simulink model "FirstOrderSystemSimulinkRL"  (R2019b)
settings: Solver=VariableStepAuto  StartTime=0.0  StopTime=25  RelTol=1e-1
values from neighbouring files (symbols this model uses):
  Ts = 0.05    [FirstOrderSystemScriptDQN.m]    (also in Trained Data Workspace.mat)
undefined symbols (not defined in the file or in its folder): DiscIntNeverNeededParam
libraries: simulink x4, dspswit3 x2, rllib x1
settings Model: Creator=PC  LastModifiedBy=PC

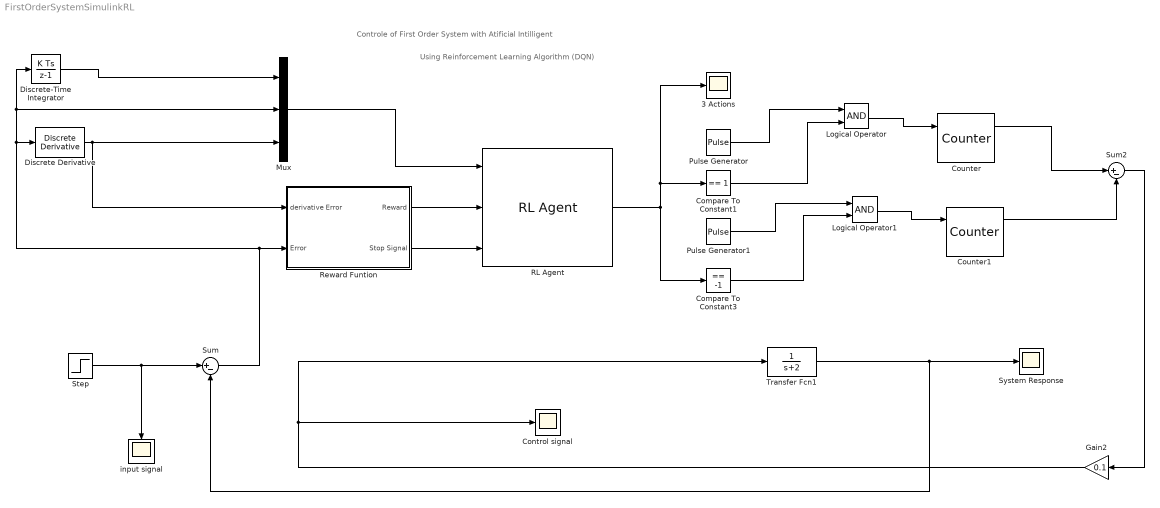
== system FirstOrderSystemSimulinkRL ==
  note: Using Reinforcement Learning Algorithm (DQN)
  note: Controle of First Order System with Atificial Intilligent
  3 Actions : Scope
  Compare To Constant1 : simulink/Logic and Bit Operations/Compare To Constant  relop===  const=1  OutDataTypeStr=boolean
  Compare To Constant3 : simulink/Logic and Bit Operations/Compare To Constant  relop===  const=-1  OutDataTypeStr=boolean
  Control signal : Scope
  Counter : dspswit3/Counter  Direction=Up  CountEvent=Rising edge  CounterSize=User defined  MaxCount=1000  InitialCount=0  Output=Count and Hit  HitValue=32  ResetInput=on  SamplesPerFrame=1  Ts=1  CntDtype=double  HitDtype=Logical
  Counter1 : dspswit3/Counter  Direction=Up  CountEvent=Rising edge  CounterSize=User defined  MaxCount=1000  InitialCount=0  Output=Count and Hit  HitValue=32  ResetInput=on  SamplesPerFrame=1  Ts=1  CntDtype=double  HitDtype=Logical
  Discrete Derivative : simulink/Discrete/Discrete Derivative  gainval=1.0  ICPrevScaledInput=0.0  OutMin=[]  OutMax=[]  OutDataType=fixdt(1, 16)  OutScaling=2^-10  DoSatur=off
  Discrete-Time Integrator : DiscreteIntegrator  SampleTime=Ts  ICPrevOutput=DiscIntNeverNeededParam  ICPrevScaledInput=DiscIntNeverNeededParam
  Gain2 : Gain  Gain=0.1
  Logical Operator : Logic  AllPortsSameDT=off  OutDataTypeStr=boolean
  Logical Operator1 : Logic  AllPortsSameDT=off  OutDataTypeStr=boolean
  Mux : Mux  Inputs=3
  Pulse Generator : DiscretePulseGenerator  PulseType=Time based  Period=0.1  PulseWidth=0.05
  Pulse Generator1 : DiscretePulseGenerator  PulseType=Time based  Period=0.1  PulseWidth=0.05
  RL Agent : rllib/RL Agent  Agent=agent  ProvideReward=on  ProvideIsDone=on  ProvideCumRwd=off  TreatAsDirectFeedthrough=on  CollectLoggedSignals=on  CollectModelStates=on
      settings: SourceProductName=Reinforcement Learning Toolbox
  Reward Funtion : Subsystem
  Step : Step  Time=0  SampleTime=0
  Sum : Sum  Inputs=|+-
  Sum2 : Sum  Inputs=|+-
  System Response : Scope
  Transfer Fcn1 : TransferFcn  Denominator=[1 2]
  input signal : Scope
  wires:
  Step/1 -> Sum/1, input signal/1
  Sum/1 -> Reward Funtion/2(Error), Discrete-Time Integrator/1, Mux/2, Discrete Derivative/1
  Discrete-Time Integrator/1 -> Mux/1
  Discrete Derivative/1 -> Reward Funtion/1(derivative Error), Mux/3
  Mux/1 -> RL Agent/1
  RL Agent/1 -> 3 Actions/1, Compare To Constant1/1, Compare To Constant3/1
  Pulse Generator/1 -> Logical Operator/1
  Logical Operator/1 -> Counter/1
  Compare To Constant1/1 -> Logical Operator/2
  Compare To Constant3/1 -> Logical Operator1/2
  Logical Operator1/1 -> Counter1/1
  Pulse Generator1/1 -> Logical Operator1/1
  Counter/1 -> Sum2/1
  Counter1/1 -> Sum2/2
  Sum2/1 -> Gain2/1
  Reward Funtion/1(Reward) -> RL Agent/2
  Reward Funtion/2(Stop Signal) -> RL Agent/3
  Gain2/1 -> Transfer Fcn1/1, Control signal/1
  Transfer Fcn1/1 -> Sum/2, System Response/1

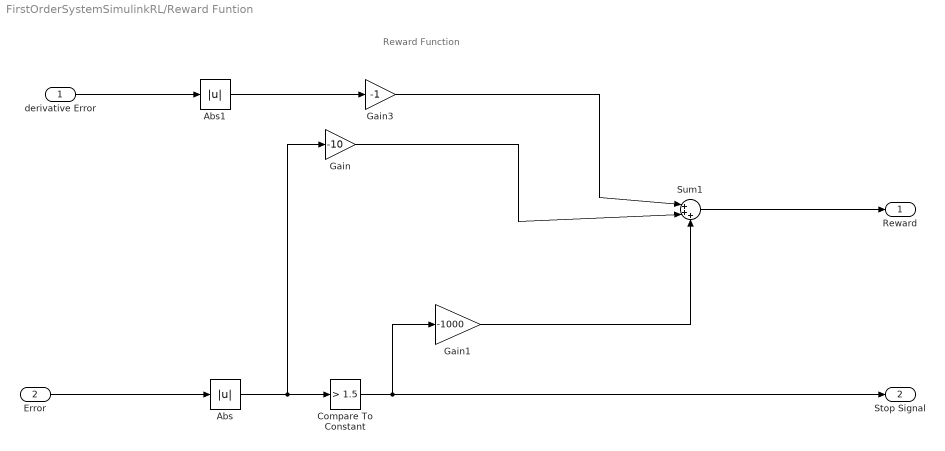
== system FirstOrderSystemSimulinkRL/Reward Funtion ==
  note: Reward Function
  derivative Error : Inport
  Error : Inport  Port=2
  Abs : Abs
  Abs1 : Abs
  Compare To Constant : simulink/Logic and Bit Operations/Compare To Constant  relop=>  const=1.5  OutDataTypeStr=boolean
  Gain : Gain  Gain=-10
  Gain1 : Gain  Gain=-1000
  Gain3 : Gain  Gain=-1
  Sum1 : Sum  Inputs=|+++
  Reward : Outport
  Stop Signal : Outport  Port=2
  wires:
  Compare To Constant/1 -> Stop Signal/1, Gain1/1
  Abs/1 -> Compare To Constant/1, Gain/1
  derivative Error/1 -> Abs1/1
  Error/1 -> Abs/1
  Abs1/1 -> Gain3/1
  Sum1/1 -> Reward/1
  Gain1/1 -> Sum1/3
  Gain/1 -> Sum1/2
  Gain3/1 -> Sum1/1
